simulink model "dyb"  (R2022b)
settings: Solver=VariableStepAuto  StartTime=0.0  StopTime=10.0  RelTol=1e-3
undefined symbols (not defined in the file): Ion, Lithium
libraries: spsDiodeLib x8, spsSeriesRLCBranchLib x5, spsVoltageMeasurementLib x5, spsCurrentMeasurementLib x4, spsIGBTDiodeLib x4, spsACVoltageSourceLib x1, spsBatteryLib x1, spsMutualInductanceLib x1, sps_lib x1
settings Model: Creator=alper  LastModifiedBy=alper
settings SolverCC: ZeroCrossAlgorithm=Adaptive
settings DebuggingCC: MaskedZcDiagnostic=none  IgnoredZcDiagnostic=none

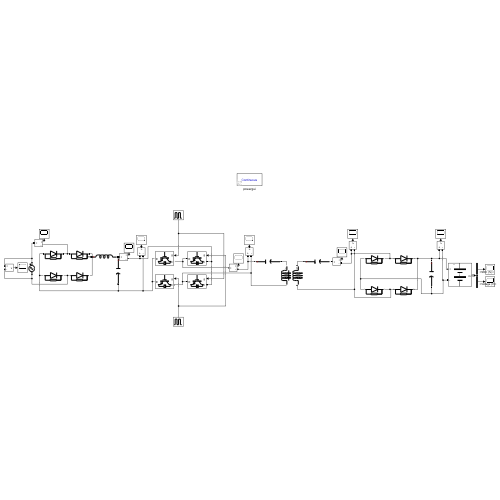
[thumbnail: Simulink's stored preview of the top-level diagram]
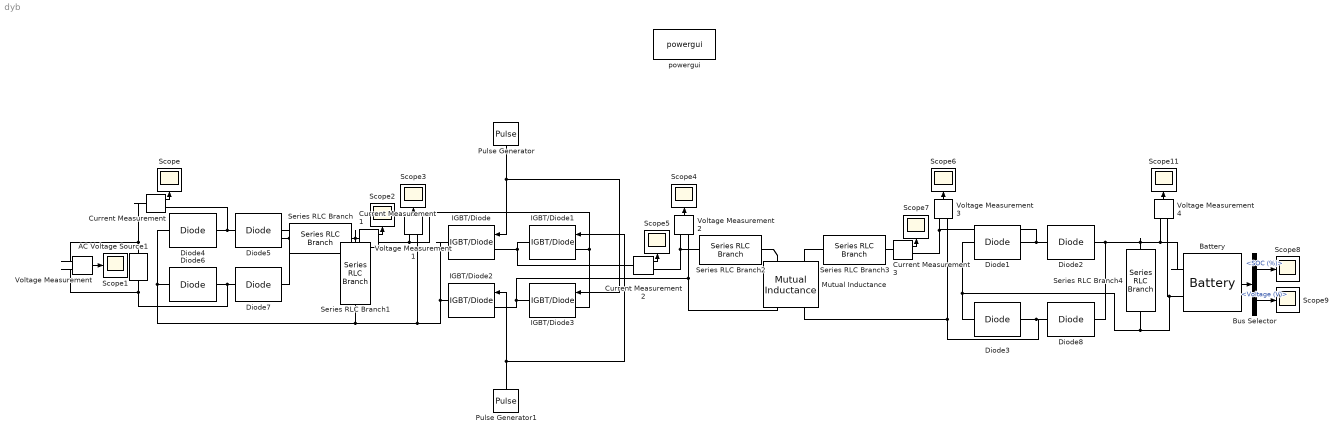
== system dyb ==
  AC Voltage Source1 : spsACVoltageSourceLib/AC Voltage Source  Amplitude=325  Phase=0  Frequency=50  SampleTime=0  Measurements=None  BusType=swing  Pref=10e3  Qref=0  Qmin=-inf  Qmax=+inf
  Battery : spsBatteryLib/Battery  BatType=Lithium-Ion  ShowTempParam=off  ThermalPreset=no  ShowAgeParam=off  NomV=180  NomQ=100  SOC=10  Batt_Tr=10  PresetModel=on  MaxQ=100  MinV=135  FullV=209.5177  Dis_rate=43.4783  R=0.018  Normal_OP=90.4348  expZone="[194.4695      4.913043]"  current=[6.5 13 32.5]  Units=Time  Tci=20  NomT=20  T2=-30  MaxQ2=4.8  FullV2=7.1  Normal_OP2=5.655  expZone2="[6.58           1]"  Rca=0.6  ti=2000  Dp=0  Neq0=0  Tsim=1e6  Ta1=25  Qeol=5.4*0.9  Reol=0.013333*1.2  Char_age=[2.3478, 3]  Dis_age=[2.3478, 10]  N1=1500  N2=10500  N3=1000  N4=1400  Ta2=45  N5=950
  Bus Selector : BusSelector  OutputSignals=SOC (%),Voltage (V)
  Current Measurement{,1..3} (4 alike) : spsCurrentMeasurementLib/Current Measurement  PhasorSimulation=off  OutputType=Complex  PSBequivalent=0
  Diode{1..8} (8 alike) : spsDiodeLib/Diode  Ron=0.001  Lon=0  Vf=0.8  IC=0  UseSnubber=0  Rs=500  Cs=250e-9  Measurements=off
  IGBT/Diode{,1..3} (4 alike) : spsIGBTDiodeLib/IGBT//Diode  Ron=1e-3  Rs=1e5  Cs=inf  Measurements=off
  Mutual Inductance : spsMutualInductanceLib/Mutual Inductance  LConnTagsString=a|b  RConnTagsString=A|B  TypeOfMutual=Two or three windings with equal mutual terms  NumberOfWindings=3  SelfImpedance1=[1e-3 266.16e-6]  SelfImpedance2=[1e-3 256.79e-6]  ThreeWindings=off  SelfImpedance3=[ 1.1 1.1e-03]  MutualImpedance=[0 85.46e-6]  InductanceMatrix="[1.0 0.9  0.9 ;  0.9 1.0  0.9;  0.9 0.9 1.0 ] * 1e-3"  ResistanceMatrix="[1.0 0.9  0.9 ;  0.9 1.0  0.9;  0.9 0.9 1.0 ]"  Measurements=None
      settings: LibrarySourceBlock=sps_lib/Passives/Mutual Inductance
  Pulse Generator : DiscretePulseGenerator  PulseType=Time based  Period=0.002  PulseWidth=50
  Pulse Generator1 : DiscretePulseGenerator  PulseType=Time based  Period=0.002  PulseWidth=50  PhaseDelay=0.001
  Scope{,1..9,11} (11 alike) : Scope
  Series RLC Branch : spsSeriesRLCBranchLib/Series RLC Branch  LConnTagsString=__new0  RConnTagsString=__new0  BranchType=L  Resistance=0  Inductance=10e-3  SetiL0=off  InitialCurrent=0  Capacitance=0  Setx0=off  InitialVoltage=0  Measurements=None
  Series RLC Branch1 : spsSeriesRLCBranchLib/Series RLC Branch  LConnTagsString=__new0  RConnTagsString=__new0  BranchType=C  Resistance=1  Inductance=1e-3  SetiL0=off  InitialCurrent=0  Capacitance=300e-6  Setx0=off  InitialVoltage=0  Measurements=None
  Series RLC Branch2 : spsSeriesRLCBranchLib/Series RLC Branch  LConnTagsString=__new0  RConnTagsString=__new0  BranchType=C  Resistance=1  Inductance=1e-3  SetiL0=off  InitialCurrent=0  Capacitance=105.74e-9  Setx0=off  InitialVoltage=0  Measurements=None
  Series RLC Branch3 : spsSeriesRLCBranchLib/Series RLC Branch  LConnTagsString=__new0  RConnTagsString=__new0  BranchType=C  Resistance=1  Inductance=1e-3  SetiL0=off  InitialCurrent=0  Capacitance=109.69e-9  Setx0=off  InitialVoltage=0  Measurements=None
  Series RLC Branch4 : spsSeriesRLCBranchLib/Series RLC Branch  LConnTagsString=__new0  RConnTagsString=__new0  BranchType=C  Resistance=1  Inductance=1e-3  SetiL0=off  InitialCurrent=0  Capacitance=300e-6  Setx0=off  InitialVoltage=0  Measurements=None
  Voltage Measurement{,1..4} (5 alike) : spsVoltageMeasurementLib/Voltage Measurement  PhasorSimulation=off  OutputType=Complex  PSBequivalent=0
  powergui : sps_lib/powergui  Priority=1  SimulationMode=Continuous  SampleTime=50e-6  frequency=60  Iterations=50  frequencyindice=50  Pbase=100e6  ErrMax=1e-4  UnitsV=kV  UnitsW=MW  buscounter=0  FunctionMessages=off  echomessages=off  EnableUseOfTLC=off  CurrentSourceSwitches=off  DisableSnubberDevices=off  DisableRonSwitches=off  DisableVfSwitches=off  DisplayEquations=off  AutomaticDiscreteSolvers=off  SolverType=Tustin/Backward Euler (TBE)  Interpol=off  ExternalGateDelay=off  methode=off  Ts=100  x0status=blocks  SPID=on  SwTol=0  HookPort=off  NonlinearTolerance=1e-4  nMaxIteration=100  ContinueOnMaxIteration=off  RestoreLinks=warning  ResistiveCurrentMeasurement=off  Frange=[0:2:500]  Ylog=off  Xlog=on  ShowGrid=off  save=off  variable=ZData  structure=0  ZoomFFT=off  StartTime=0.0  cycles=1  DisplayStyle=1  fundamental=60  FreqAxis=off  MaxFrequency=1000  frequencyindicesteady=1  RmsSteady=1  display=off
  wires:
  Current Measurement/1 -> Scope/1
  Voltage Measurement/1 -> Scope1/1
  Current Measurement1/1 -> Scope2/1
  Voltage Measurement1/1 -> Scope3/1
  Voltage Measurement2/1 -> Scope4/1
  Pulse Generator/1 -> IGBT/Diode/1, IGBT/Diode3/1
  Pulse Generator1/1 -> IGBT/Diode1/1, IGBT/Diode2/1
  Current Measurement2/1 -> Scope5/1
  Current Measurement3/1 -> Scope7/1
  Voltage Measurement3/1 -> Scope6/1
  Battery/1 -> Bus Selector/1
  Bus Selector/1 -> Scope8/1  "<SOC (%)>"
  Bus Selector/2 -> Scope9/1  "<Voltage (V)>"
  Voltage Measurement4/1 -> Scope11/1
  connections:
  Diode4/RConn1 -- Current Measurement/RConn1 -- Diode5/LConn1
  AC Voltage Source1/LConn1 -- Diode7/LConn1 -- Diode6/RConn1 -- Voltage Measurement/LConn2
  Diode5/RConn1 -- Diode7/RConn1 -- Series RLC Branch/LConn1
  Current Measurement/LConn1 -- Voltage Measurement/LConn1 -- AC Voltage Source1/RConn1
  Diode4/LConn1 -- Diode6/LConn1 -- Series RLC Branch1/RConn1 -- IGBT/Diode2/RConn1 -- IGBT/Diode/RConn1 -- Voltage Measurement1/LConn2
  Series RLC Branch/RConn1 -- Series RLC Branch1/LConn1 -- Current Measurement1/LConn1
  Current Measurement1/RConn1 -- IGBT/Diode3/LConn1 -- IGBT/Diode1/LConn1 -- Voltage Measurement1/LConn1
  IGBT/Diode2/LConn1 -- Mutual Inductance/RConn1 -- Voltage Measurement2/LConn2 -- IGBT/Diode3/RConn1
  IGBT/Diode/LConn1 -- Current Measurement2/LConn1 -- IGBT/Diode1/RConn1
  Current Measurement2/RConn1 -- Series RLC Branch2/LConn1 -- Voltage Measurement2/LConn1
  Mutual Inductance/RConn2 -- Diode8/LConn1 -- Diode3/RConn1 -- Voltage Measurement3/LConn2
  Mutual Inductance/LConn2 -- Series RLC Branch3/LConn1
  Series RLC Branch2/RConn1 -- Mutual Inductance/LConn1
  Series RLC Branch3/RConn1 -- Current Measurement3/LConn1
  Current Measurement3/RConn1 -- Diode1/RConn1 -- Diode2/LConn1 -- Voltage Measurement3/LConn1
  Diode3/LConn1 -- Diode1/LConn1 -- Voltage Measurement4/LConn2 -- Battery/LConn2 -- Series RLC Branch4/RConn1
  Diode2/RConn1 -- Series RLC Branch4/LConn1 -- Battery/LConn1 -- Voltage Measurement4/LConn1 -- Diode8/RConn1
